simulink model "Model_Test"  (R2019b)
settings: Solver=VariableStepAuto  StartTime=0.0  StopTime=10.0  RelTol=1e-3
undefined symbols (not defined in the file or in its folder): i
settings Model: Creator=uic26460  LastModifiedBy=uic26460

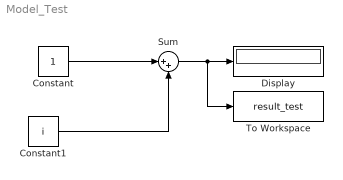
== system Model_Test ==
  Constant : Constant
  Constant1 : Constant  Value=i
  Display : Display
  Sum : Sum  Inputs=|++
  To Workspace : ToWorkspace  VariableName=result_test  SaveFormat=Timeseries  SampleTime=-1
  wires:
  Constant/1 -> Sum/1
  Sum/1 -> To Workspace/1, Display/1
  Constant1/1 -> Sum/2
